simulink model "SimulinkEx2"  (R2024a)
settings: Solver=ode4  StartTime=0.0  StopTime=10.0  FixedStep=0.01  RelTol=1e-3
values from neighbouring files (symbols this model uses):
  Ae = [A, zeros(2,1) ... (first row only)    [Ex2.m]
  Be = [B; 0]    [Ex2.m]
  Ce = [C, 0]    [Ex2.m]
  Gcon = minreal(K/(s*eye(2) - (A-B*K-Ke*C))*Ke,1e-4)    [Ex2.m]
settings Model: Creator=caugu  LastModifiedBy=caugu

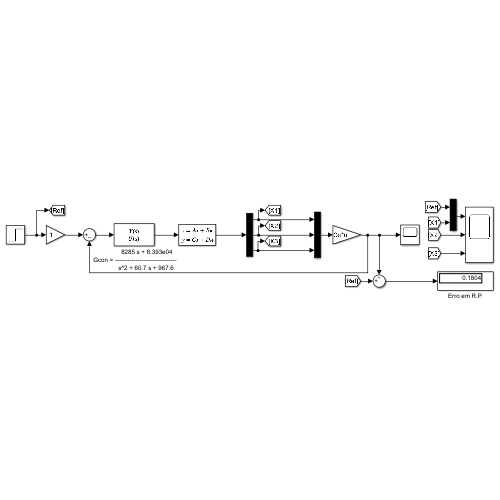
[thumbnail: Simulink's stored preview of the top-level diagram]
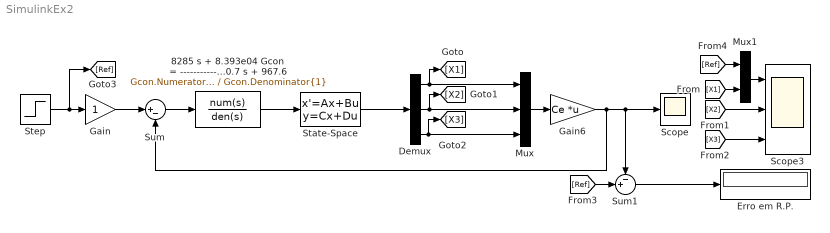
== system SimulinkEx2 ==
  "               8285 s + 8.393e04 Gcon = ------------------------------ s^2 + 60.7 s + 967.6" : TransferFcn  Numerator=Gcon.Numerator{1}  Denominator=Gcon.Denominator{1}
  Demux : Demux  Outputs=3
  Erro em R.P. : Display
  Gain : Gain
  Gain6 : Gain  Gain=Ce  Multiplication=Matrix(K*u)
  Mux : Mux  Inputs=3
  Mux1 : Mux  Inputs=2
  Scope : Scope
  Scope3 : Scope  NumInputPorts=3
  State-Space : StateSpace  A=Ae  B=Be  C=eye(3)  D=zeros(3,1)  InitialCondition=0
  Step : Step  Time=0  SampleTime=0
  Sum : Sum  Inputs=|+-
  Sum1 : Sum  Inputs=-+|
  wires:
  Demux/1 -> [X1], Mux/1
  Gain6/1 -> Scope/1, Sum1/1, Sum/2
  Mux/1 -> Gain6/1
  Demux/2 -> [X2], Mux/2
  State-Space/1 -> Demux/1
  Gain/1 -> Sum/1
  Demux/3 -> [X3], Mux/3
  Sum/1 -> "               8285 s + 8.393e04 Gcon = ------------------------------ s^2 + 60.7 s + 967.6"/1
  "               8285 s + 8.393e04 Gcon = ------------------------------ s^2 + 60.7 s + 967.6"/1 -> State-Space/1
  Step/1 -> [Ref], Gain/1
  Sum1/1 -> Erro em R.P./1
  [X2] -> Scope3/2
  [X3] -> Scope3/3
  [Ref] -> Sum1/2
  [X1] -> Mux1/2
  [Ref] -> Mux1/1
  Mux1/1 -> Scope3/1
